simulink model "Modified_HDL_Counter"  (R2019b)
settings: Solver=VariableStepAuto  StartTime=0.0  StopTime=10.0  RelTol=1e-3
undefined symbols (not defined in the file or in its folder): CountFracLen, CountFrom, CountInit, CountWordLen, freerun, issigned, maxval_sc, samptime
libraries: hdlsllib x3, simulink x1
settings Model: Creator=larry  LastModifiedBy=larry

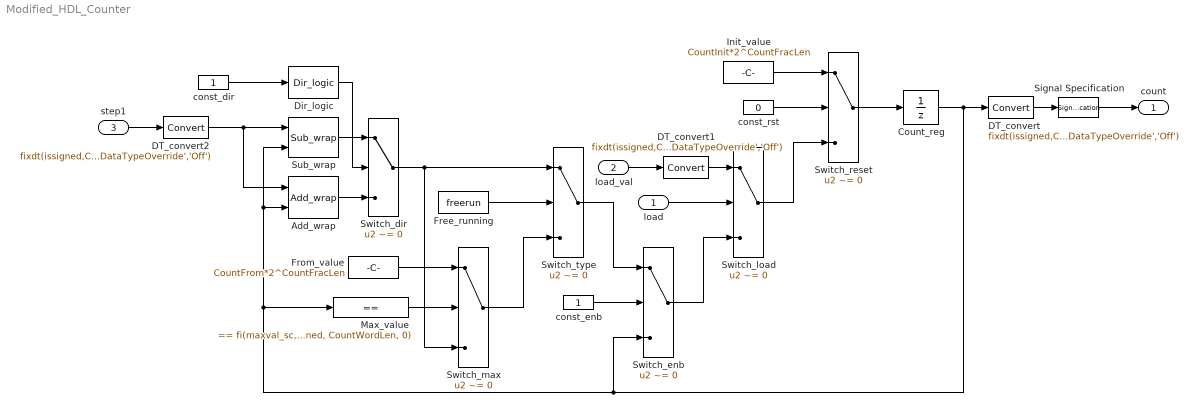
== system Modified_HDL_Counter ==
  load : Inport  OutDataTypeStr=boolean  PortDimensions=1
  load_val : Inport  Port=2  OutDataTypeStr=fixdt(issigned,CountWordLen,CountFracLen,'DataTypeOverride','Off')  PortDimensions=1
  step1 : Inport  Port=3  OutDataTypeStr=fixdt(issigned,CountWordLen,CountFracLen,'DataTypeOverride','Off')  PortDimensions=1
  Add_wrap : hdlsllib/Sources/HDL Counter/Add_wrap  SystemSampleTime=-1  Latency=0  AutoFrameSizeCalculation=off
      settings: SourceProductName=Simulink  SourceProductBaseCode=SL
  Count_reg : UnitDelay  InitialCondition=CountInit*2^CountFracLen  SampleTime=samptime  HasFrameUpgradeWarning=on
  DT_convert : DataTypeConversion  OutDataTypeStr=fixdt(issigned,CountWordLen,CountFracLen,'DataTypeOverride','Off')  ConvertRealWorld=Stored Integer (SI)
  DT_convert1 : DataTypeConversion  OutDataTypeStr=fixdt(issigned,CountWordLen,0,'DataTypeOverride','Off')  ConvertRealWorld=Stored Integer (SI)
  DT_convert2 : DataTypeConversion  OutDataTypeStr=fixdt(issigned,CountWordLen,0,'DataTypeOverride','Off')  ConvertRealWorld=Stored Integer (SI)
  Dir_logic : hdlsllib/Sources/HDL Counter/Dir_logic  SystemSampleTime=-1  Latency=0  AutoFrameSizeCalculation=off
      settings: SourceProductName=Simulink  SourceProductBaseCode=SL
  Free_running : Constant  Value=freerun  OutDataTypeStr=boolean
  From_value : Constant  Value=CountFrom*2^CountFracLen  OutDataTypeStr=fixdt(issigned,CountWordLen, 0,'DataTypeOverride','Off')
  Init_value : Constant  Value=CountInit*2^CountFracLen  OutDataTypeStr=fixdt(issigned,CountWordLen, 0,'DataTypeOverride','Off')
  Max_value : simulink/Logic and Bit Operations/Compare To Constant  relop===  const=fi(maxval_sc, issigned, CountWordLen, 0)  OutDataTypeStr=boolean  ZeroCross=off
  Signal Specification : SignalSpecification  Dimensions=1
  Sub_wrap : hdlsllib/Sources/HDL Counter/Sub_wrap  SystemSampleTime=-1  Latency=0  AutoFrameSizeCalculation=off
      settings: SourceProductName=Simulink  SourceProductBaseCode=SL
  Switch_dir : Switch  Criteria=u2 ~= 0
  Switch_enb : Switch  Criteria=u2 ~= 0
  Switch_load : Switch  Criteria=u2 ~= 0
  Switch_max : Switch  Criteria=u2 ~= 0
  Switch_reset : Switch  Criteria=u2 ~= 0  OutDataTypeStr=fixdt(issigned,CountWordLen, 0,'DataTypeOverride','Off')
  Switch_type : Switch  Criteria=u2 ~= 0
  const_dir : Constant  OutDataTypeStr=boolean
  const_enb : Constant  OutDataTypeStr=boolean
  const_rst : Constant  Value=0  OutDataTypeStr=boolean
  count : Outport  VectorParamsAs1DForOutWhenUnconnected=off
  wires:
  Switch_load/1 -> Switch_reset/3
  Max_value/1 -> Switch_max/2
  Switch_reset/1 -> Count_reg/1
  Sub_wrap/1 -> Switch_dir/1
  Add_wrap/1 -> Switch_dir/3
  Switch_dir/1 -> Switch_type/1, Switch_max/3
  step1/1 -> DT_convert2/1
  const_rst/1 -> Switch_reset/2
  DT_convert2/1 -> Add_wrap/1, Sub_wrap/1
  Free_running/1 -> Switch_type/2
  DT_convert/1 -> Signal Specification/1
  const_enb/1 -> Switch_enb/2
  const_dir/1 -> Dir_logic/1
  Switch_enb/1 -> Switch_load/3
  load/1 -> Switch_load/2
  Init_value/1 -> Switch_reset/1
  Signal Specification/1 -> count/1
  Dir_logic/1 -> Switch_dir/2
  From_value/1 -> Switch_max/1
  load_val/1 -> DT_convert1/1
  Switch_type/1 -> Switch_enb/1
  Switch_max/1 -> Switch_type/3
  Count_reg/1 -> Switch_enb/3, Max_value/1, Sub_wrap/2, Add_wrap/2, DT_convert/1
  DT_convert1/1 -> Switch_load/1
